simulink model "plant_simscape"  (R2023b)
settings: Solver=VariableStepAuto  StartTime=0.0  StopTime=10.0  RelTol=1e-3
undefined symbols (not defined in the file or in its folder): param, x0
libraries: fl_lib x15, nesl_utility x7
settings Model: Creator=block  LastModifiedBy=block

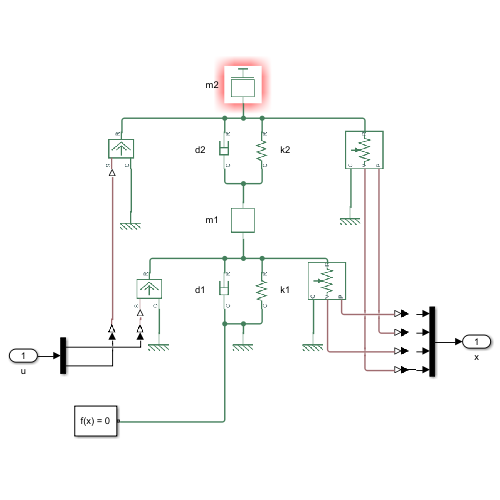
[thumbnail: Simulink's stored preview of the top-level diagram]
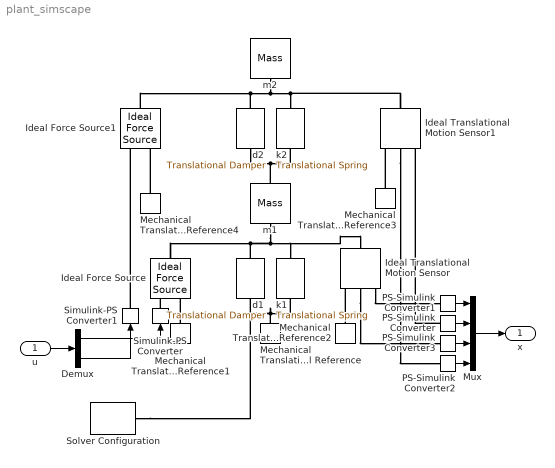
== system plant_simscape ==
  u : Inport
  Demux : Demux  Outputs=2
  Ideal Force Source : fl_lib/Mechanical/Mechanical Sources/Ideal Force Source
  Ideal Force Source1 : fl_lib/Mechanical/Mechanical Sources/Ideal Force Source
  Ideal Translational Motion Sensor : fl_lib/Mechanical/Mechanical Sensors/Ideal Translational Motion Sensor  reference=foundation.enum.MeasurementReference.difference  acceleration_port=false  velocity_port=true  position_port=true  offset=x0(1) m
  Ideal Translational Motion Sensor1 : fl_lib/Mechanical/Mechanical Sensors/Ideal Translational Motion Sensor  reference=foundation.enum.MeasurementReference.difference  acceleration_port=false  velocity_port=true  position_port=true  offset=x0(2) m
  Mechanical Translational Reference{,1..4} (5 alike) : fl_lib/Mechanical/Translational Elements/Mechanical Translational Reference
  Mux : Mux
  PS-Simulink Converter{,1..3} (4 alike) : nesl_utility/PS-Simulink Converter  PhysicalDomain=network_engine_domain  SubClassName=ps_output  LeftPortType=input  RightPortType=output  PseudoPeriodic=off  Frequencies=[]  VectorFormat=inherit  Unit=inherit  AffineConversion=off
  Simulink-PS Converter : nesl_utility/Simulink-PS Converter  PhysicalDomain=network_engine_domain  SubClassName=ps_input  LeftPortType=input  RightPortType=output  PseudoPeriodic=off  Frequencies=[]  NoiseDistribution=none  NoiseParameters=[]  Unit=1  AffineConversion=off  FilteringAndDerivatives=provide  SimscapeFilterOrder=1  InputFilterTimeConstant=0.001  UdotUserProvided=0
  Simulink-PS Converter1 : nesl_utility/Simulink-PS Converter  PhysicalDomain=network_engine_domain  SubClassName=ps_input  LeftPortType=input  RightPortType=output  PseudoPeriodic=off  Frequencies=[]  NoiseDistribution=none  NoiseParameters=[]  Unit=1  AffineConversion=off  FilteringAndDerivatives=provide  SimscapeFilterOrder=1  InputFilterTimeConstant=0.001  UdotUserProvided=0
  Solver Configuration : nesl_utility/Solver Configuration  PhysicalDomain=network_engine_domain  SubClassName=solver  LeftPortType=input  RightPortType=generic  Tones=[]  Harmonics=[]  SimulateNoise=off  Profile=off  UseLocalSampling=off  EnableSwitchedLinearOptims=on  FrequencyDomain=off  UseCCode=off  RelTol=0.001  AbsTol=0.001  MinStep=1e-09  ToWorkspace=off  RevertToSquareIcSolve=off  NumHomotopyIterations=100  PhasorMode=off  PhasorModeNumHarmonics=1  ConsistencySolver=NEWTON_XTOL_AFTER_FTOL  IndexReductionMethod=DerivativeReplacement  DoDC=off  ResidualTolerance=1e-09  ConsistencyTolSource=GLOBAL  ConsistencyAbsTol=0.001  ConsistencyRelTol=0.001  ConsistencyTolFactor=0.001  UseLocalSolver=off  LocalSolverChoice=NE_BACKWARD_EULER_ADVANCER  ResolveIndetEquations=on  FunctionEvalNumThread=1  LocalSolverSampleTime=0.001  DoFixedCost=off  MaxNonlinIter=3  MaxModeIter=2  ComputeImpulses=off  ImpulseIterations=2  LinearAlgebra=auto  LinearAlgebraNumThread=0  EquationFormulation=NE_TIME_EF  DelaysMemoryBudget=1024  AutomaticFiltering=on  FilteringTimeConstant=0.001  PartitionStorageMethod=AS_NEEDED  PartitionMemoryBudget=1024  PartitionMethod=ROBUST  MultibodyUseLocalSolver=off  MultibodyLocalSolverChoice=ODE1  MultibodyLocalSolverSampleTime=0.001
  d1 : fl_lib/Mechanical/Translational Elements/Translational Damper  D=param.d1 N*s/m  v_specify=off  v_priority=None  v=0 m/s  v_nominal_specify=off  v_nominal_unit=m/s  v_nominal_value=1  f_specify=off  f_priority=None  f=0 N  f_nominal_specify=off  f_nominal_unit=N  f_nominal_value=1
  d2 : fl_lib/Mechanical/Translational Elements/Translational Damper  D=param.d2 N*s/m  v_specify=off  v_priority=None  v=0 m/s  v_nominal_specify=off  v_nominal_unit=m/s  v_nominal_value=1  f_specify=off  f_priority=None  f=0 N  f_nominal_specify=off  f_nominal_unit=N  f_nominal_value=1
  k1 : fl_lib/Mechanical/Translational Elements/Translational Spring  spr_rate=param.k1 N/m  v_specify=off  v_priority=None  v=x0(2) m/s  v_nominal_specify=off  v_nominal_unit=m/s  v_nominal_value=1  f_specify=off  f_priority=None  f=0 N  f_nominal_specify=off  f_nominal_unit=N  f_nominal_value=1  x_specify=on  x_priority=High  x=x0(1) m  x_nominal_specify=off  x_nominal_unit=m  x_nominal_value=1
  k2 : fl_lib/Mechanical/Translational Elements/Translational Spring  spr_rate=param.k2 N/m  v_specify=off  v_priority=None  v=x0(2) m/s  v_nominal_specify=off  v_nominal_unit=m/s  v_nominal_value=1  f_specify=off  f_priority=None  f=0 N  f_nominal_specify=off  f_nominal_unit=N  f_nominal_value=1  x_specify=on  x_priority=High  x=x0(2)-x0(1) m  x_nominal_specify=off  x_nominal_unit=m  x_nominal_value=1
  m1 : fl_lib/Mechanical/Translational Elements/Mass  mass=param.m1 kg  num_ports=foundation.enum.numPorts2.two  v_specify=on  v_priority=High  v=x0(3) m/s  v_nominal_specify=off  v_nominal_unit=m/s  v_nominal_value=1  f_specify=off  f_priority=None  f=0 N  f_nominal_specify=off  f_nominal_unit=N  f_nominal_value=1
      settings: InternalSimscapePortConfiguration="{\"Bottom\":[],\"Left\":[{\"id\":\"M\",\"label\":\"\",\"type\":\"foundation.mechanical.translational.translational\"}],\"Right\":[{\"id\":\"N\",\"label\":\"\",\"type\":\"foundation.mechanical.translational.translational\"}],\"Top\":[]}"
  m2 : fl_lib/Mechanical/Translational Elements/Mass  mass=param.m2 kg  num_ports=foundation.enum.numPorts2.one  v_specify=on  v_priority=High  v=x0(4) m/s  v_nominal_specify=off  v_nominal_unit=m/s  v_nominal_value=1  f_specify=off  f_priority=None  f=0 N  f_nominal_specify=off  f_nominal_unit=N  f_nominal_value=1
  x : Outport
  wires:
  Demux/1 -> Simulink-PS Converter/1
  PS-Simulink Converter/1 -> Mux/2
  PS-Simulink Converter1/1 -> Mux/1
  Mux/1 -> x/1
  PS-Simulink Converter3/1 -> Mux/3
  PS-Simulink Converter2/1 -> Mux/4
  u/1 -> Demux/1
  Demux/2 -> Simulink-PS Converter1/1
  connections:
  Mechanical Translational Reference/LConn1 -- Solver Configuration/RConn1 -- d1/RConn1 -- k1/RConn1
  d1/LConn1 -- Ideal Force Source/LConn1 -- Ideal Translational Motion Sensor/LConn1 -- k1/LConn1 -- m1/LConn1
  Mechanical Translational Reference1/LConn1 -- Ideal Force Source/RConn2
  Simulink-PS Converter/RConn1 -- Ideal Force Source/RConn1
  Ideal Translational Motion Sensor/RConn2 -- PS-Simulink Converter3/LConn1
  Mechanical Translational Reference2/LConn1 -- Ideal Translational Motion Sensor/RConn1
  Ideal Translational Motion Sensor/RConn3 -- PS-Simulink Converter1/LConn1
  d2/RConn1 -- m1/RConn1 -- k2/RConn1
  d2/LConn1 -- Ideal Force Source1/LConn1 -- m2/LConn1 -- Ideal Translational Motion Sensor1/LConn1 -- k2/LConn1
  Mechanical Translational Reference3/LConn1 -- Ideal Translational Motion Sensor1/RConn1
  Ideal Translational Motion Sensor1/RConn2 -- PS-Simulink Converter2/LConn1
  PS-Simulink Converter/LConn1 -- Ideal Translational Motion Sensor1/RConn3
  Simulink-PS Converter1/RConn1 -- Ideal Force Source1/RConn1
  Mechanical Translational Reference4/LConn1 -- Ideal Force Source1/RConn2
